simulink model "SIM_EXO_DAL_MN"  (R2021b)
settings: Solver=VariableStepAuto  StartTime=0.0  StopTime=60  FixedStep=0.0001  RelTol=1e-4
undefined symbols (not defined in the file): b, dq, q, X, Y, Z
libraries: sm_lib x47, nesl_utility x7
(part 4 of 24)

== matlab function SIM_EXO_DAL_MN/PID(LGR)/MATLAB Function ==
  data: H input; ts input; b input; Kp output; Kd output; Ki output
function [Kp, Kd, Ki] = ganancias(H,ts,b)
Kp = zeros(6,1);
Kd = zeros(6,1);
Ki = zeros(6,1);

wn = 6/ts;
lambda = 10*wn;

for i = 1:6
    Kp(i) = H(i,i)*(wn^2+2*wn*lambda);
    Kd(i) = H(i,i)*(lambda + 2*(wn^2))-b(i);
    Ki(i) = H(i,i)*(wn^2)*lambda;
end

== matlab function SIM_EXO_DAL_MN/PID(LGR)/MATLAB Function1 ==
  data: Kp input; tau output; Kd input; Ki input; e input; e_int input; dq input
function tau = PID(Kp,Kd,Ki,e,e_int,dq)
    tau = Kp.*e - Kd.*dq + Ki.*e_int;
